simulink library "NeuroMuscularLibrary"  (R2019b)
settings: Solver=ode45  StartTime=0.0  StopTime=10.0  RelTol=1e-3  EnableMultiTasking=on
values from neighbouring files (symbols this model uses):
  a_18_19 = 116    [Prosthesis3R60Params.m]
  a_18_21 = 34    [Prosthesis3R60Params.m]
  a_2_3 = 18    [Prosthesis3R60Params.m]
  angle_offset = 0    [Prosthesis3R60Params.m]
  ankle_height = 0.08    [BodyMechParams.m]
  c = 0.05    [BodyMechParams.m]
  c_jointstop = 0.3 / (pi/180)    (= 17.1887338539)    [BodyMechParams.m]
  c_stance_comp_a0 = 885.0653    [Prosthesis3R60Params.m]
  c_stance_comp_a1 = 2.1443    [Prosthesis3R60Params.m]
  cg14 = 1/2*L14    (= 0.0475)    [Prosthesis3R60Params.m]
  cg25 = (5.45/11.05)*L25    (= 0.0379527149321)    [Prosthesis3R60Params.m]
  cg3 = (3.6/10.4)*L3    (= 0.0306346153846)    [Prosthesis3R60Params.m]
  d_fBall = 0.1    [BodyMechParams.m]
  d_fHeel = 0.05    [BodyMechParams.m]
  deltaLegAngleThr = 8*pi/180    (= 0.13962634016)    [CMGParams.m]
  DeltaThRef = 2e-3    (= 0.002)    [BodyMechParams.m]
  dt_visual = 0.001    [Prosthesis3R60Params.m]
  eref = 0.04    [BodyMechParams.m]
  Fmax = 4000    [MuscleEnergyTest.m]
  FmaxGLU = 1500    [BodyMechParams.m]
  footBallToAnkleDist = 0.16    [BodyMechParams.m]
  footBallToCenterDist = footLength/2    (= 0.1)    [BodyMechParams.m]
  footBallToHeelDist = footLength    (= 0.2)    [BodyMechParams.m]
  footCenterToCGDist = 0.14 - footBallToCenterDist    (= 0.04)    [BodyMechParams.m]
  footInertia = 0.005    [BodyMechParams.m]
  footLength = 0.2    [BodyMechParams.m]
  footMass = 1.25    [BodyMechParams.m]
  FT = 20    [MuscleEnergyTest.m]
  FT_GLU = 47.6    [BodyMechParams.m]
  g = 9.80665    [BodyMechParams.m]
  groundTheta = [atan(diff(groundZ)./diff(groundX)), 0]    [generateGround.m]
  groundZ = groundZ * stepSize/(largestStep+eps)    [generateGround.m]
  hatCenterToCGDist = 0.35 - hatHipToCenterDistLen    (= -0.05)    [BodyMechParams.m]
  hatHipToCenterDistLen = hatLength/2    (= 0.4)    [BodyMechParams.m]
  hatInertia = 3    [BodyMechParams.m]
  hatLeftHipToCenterDistWidth = .15    (= 0.15)    [BodyMechParams.m]
  hatLength = 0.8    [BodyMechParams.m]
  hatMass = 53.5    [BodyMechParams.m]
  hatThickness = 0.2    [BodyMechParams.m]
  hatWidth = 0.4    [BodyMechParams.m]
  J1011 = (4130)*1e-9    (= 4.13e-06)    [Prosthesis3R60Params.m]
  J1415 = (1.18*1e5)*1e-9    (= 0.000118)    [Prosthesis3R60Params.m]
  J18192021 = (6.86*1e4)*1e-9    (= 6.86e-05)    [Prosthesis3R60Params.m]
  J2526 = (3.59*1e4)*1e-9    (= 3.59e-05)    [Prosthesis3R60Params.m]
  J3467 = (25.96*1e4)*1e-9    (= 0.0002596)    [Prosthesis3R60Params.m]
  K = 5    [BodyMechParams.m]
  k_gn = k_gn/2    (= 39226.6)    [BodyMechParams.m]
  k_gt = k_gt/2    (= 39226.6)    [BodyMechParams.m]
  k_pressure = hatMass * g / DeltaThRef    (= 262327.8875)    [BodyMechParams.m]
  k_stance = 130000    [Prosthesis3R60Params.m]
  k_swing = 18750    [Prosthesis3R60Params.m]
  L0_stance = 0.08925    [Prosthesis3R60Params.m]
  L0_swing = 0.0896    [Prosthesis3R60Params.m]
  L10 = 7.9*1e-3    (= 0.0079)    [Prosthesis3R60Params.m]
  L11 = 3.3*1e-3    (= 0.0033)    [Prosthesis3R60Params.m]
  L14 = 95*1e-3    (= 0.095)    [Prosthesis3R60Params.m]
  L15 = 8.2*1e-3    (= 0.0082)    [Prosthesis3R60Params.m]
  L18 = 25.1*1e-3    (= 0.0251)    [Prosthesis3R60Params.m]
  L19 = 17.7*1e-3    (= 0.0177)    [Prosthesis3R60Params.m]
  L20 = 26*1e-3    (= 0.026)    [Prosthesis3R60Params.m]
  L21 = 1.7*1e-3    (= 0.0017)    [Prosthesis3R60Params.m]
  L25 = 76.95*1e-3    (= 0.07695)    [Prosthesis3R60Params.m]
  L26 = 2.8*1e-3    (= 0.0028)    [Prosthesis3R60Params.m]
  L3 = 88.5*1e-3    (= 0.0885)    [Prosthesis3R60Params.m]
  L4 = 1.7*1e-3    (= 0.0017)    [Prosthesis3R60Params.m]
  L6 = 40.25*1e-3    (= 0.04025)    [Prosthesis3R60Params.m]
  L7 = 14.9*1e-3    (= 0.0149)    [Prosthesis3R60Params.m]
  leg_l = [(thighLength - ankle_height/2) (shankLength - ankle_height/2)]    [BodyMechParams.m]
  legAngleSpeedMax = 10    [CMGParams.m]
  lopt = 0.055    [MuscleEnergyTest.m]
  loptBFSH = 0.12    [BodyMechParams.m]
  loptGAS = 0.05    [BodyMechParams.m]
  loptGLU = 0.11    [BodyMechParams.m]
  loptHAB = 0.09    [BodyMechParams.m]
  loptHAD = 0.10    (= 0.1)    [BodyMechParams.m]
  loptHAM = 0.10    (= 0.1)    [BodyMechParams.m]
  loptHFL = 0.11    [BodyMechParams.m]
  loptRF = 0.08    [BodyMechParams.m]
  loptSOL = 0.04    [BodyMechParams.m]
  loptTA = 0.06    [BodyMechParams.m]
  loptVAS = 0.08    [BodyMechParams.m]
  lslack = 0.245    [MuscleEnergyTest.m]
  lslackBFSH = 0.10    (= 0.1)    [BodyMechParams.m]
  lslackGAS = 0.40    (= 0.4)    [BodyMechParams.m]
  lslackGLU = 0.13    [BodyMechParams.m]
  lslackHAB = 0.07    [BodyMechParams.m]
  lslackHAD = 0.18    [BodyMechParams.m]
  lslackHAM = 0.31    [BodyMechParams.m]
  lslackHFL = 0.10    (= 0.1)    [BodyMechParams.m]
  lslackRF = 0.35    [BodyMechParams.m]
  lslackSOL = 0.26    [BodyMechParams.m]
  lslackTA = 0.24    [BodyMechParams.m]
  lslackVAS = 0.23    [BodyMechParams.m]
  m1011 = 49.5*1e-3    (= 0.0495)    [Prosthesis3R60Params.m]
  m1415 = 123.8*1e-3    (= 0.1238)    [Prosthesis3R60Params.m]
  m18192021 = 196.6*1e-3    (= 0.1966)    [Prosthesis3R60Params.m]
  m2526 = 58.3*1e-3    (= 0.0583)    [Prosthesis3R60Params.m]
  m3467 = 253.3*1e-3    (= 0.2533)    [Prosthesis3R60Params.m]
  mu_slide = 0.8    [BodyMechParams.m]
  mu_stick = 0.9    [BodyMechParams.m]
  N = 1.5    [BodyMechParams.m]    (also in cmaes.m = size(x,1); mergeCompareEnergyCosts.m = {S.name})
  phiKneeUpLimit = 5*pi/180    (= 0.0872664625997)    [BodyMechParams.m]
  phimaxGASa = (100-90)*pi/180    (= 0.174532925199)    [BodyMechParams.m]
  phimaxGASk = (180-140)*pi/180    (= 0.698131700798)    [BodyMechParams.m]
  phimaxRFk = (180-165)*pi/180    (= 0.261799387799)    [BodyMechParams.m]
  phimaxSOL = (100-90)*pi/180    (= 0.174532925199)    [BodyMechParams.m]
  phimaxTA = (80-90)*pi/180    (= -0.174532925199)    [BodyMechParams.m]
  phimaxVAS = (180-165)*pi/180    (= 0.261799387799)    [BodyMechParams.m]
  phirefBFSH = (180-160)*pi/180    (= 0.349065850399)    [BodyMechParams.m]
  phirefGASa = (80-90)*pi/180    (= -0.174532925199)    [BodyMechParams.m]
  phirefGASk = (180-165)*pi/180    (= 0.261799387799)    [BodyMechParams.m]
  phirefGLU = (120-180)*pi/180    (= -1.0471975512)    [BodyMechParams.m]
  phirefHAB = 10*pi/180    (= 0.174532925199)    [BodyMechParams.m]
  phirefHAD = 15*pi/180    (= 0.261799387799)    [BodyMechParams.m]
  phirefHAMh = (150-180)*pi/180    (= -0.523598775598)    [BodyMechParams.m]
  phirefHAMk = (180-180)*pi/180    (= 0)    [BodyMechParams.m]
  phirefHFL = (160-180)*pi/180    (= -0.349065850399)    [BodyMechParams.m]
  phirefRFh = (170-180)*pi/180    (= -0.174532925199)    [BodyMechParams.m]
  phirefRFk = (180-125)*pi/180    (= 0.959931088597)    [BodyMechParams.m]
  phirefSOL = (90-90)*pi/180    (= 0)    [BodyMechParams.m]
  ... (+64 more)
undefined symbols (not defined in the file or in its folder): ankleBackDriveGain, ankleCJointstop, ankleDgain, ankleFilterPID, ankleFilterSEA, ankleGearEff, ankleGearRatio, ankleIgain, ankleInitialAngle, ankleInputMass, ankleIntCoulomb, ankleIntDamping, ankleIntStatic, ankleParallelSpringDamping, ankleParallelSpringOffset, ankleParallelSpringStiffness, anklePgain, anklePlantarLimit, ankleSEADamping, ankleSEAStiffness, ankleTendonMass, ankleWMaxJointstop, D12_F, D12_S, D12_T, D12z_T, D13_F, D1G_F, D1G_HAT, D1G_S, D1G_T, D1Gy_F, DeltaS, DeltaSGLU, DeltaSHFL, dryFrictionDamping, dryFrictionStiffness, dryFrictionVelThresh, footMassp, FourBarL1, FourBarL3, GainDphiHATGLUst, GainDphiHATHABst, GainDphiHATHADst, GainDphiHATHFLst, GainFGASst, GainFGLUst, GainFHABst, GainFHAMst, GainFSOLst, GainFSOLTAst, GainFVASst, GainGAS, GainGLU, GainGLUswing, GainHAM, GainHAMHFL ... (+194)
libraries: sm_lib x332, nesl_utility x156, simulink x33, dspswit3 x30, $bdroot x19, simulink_extras x7
(part 4 of 15)

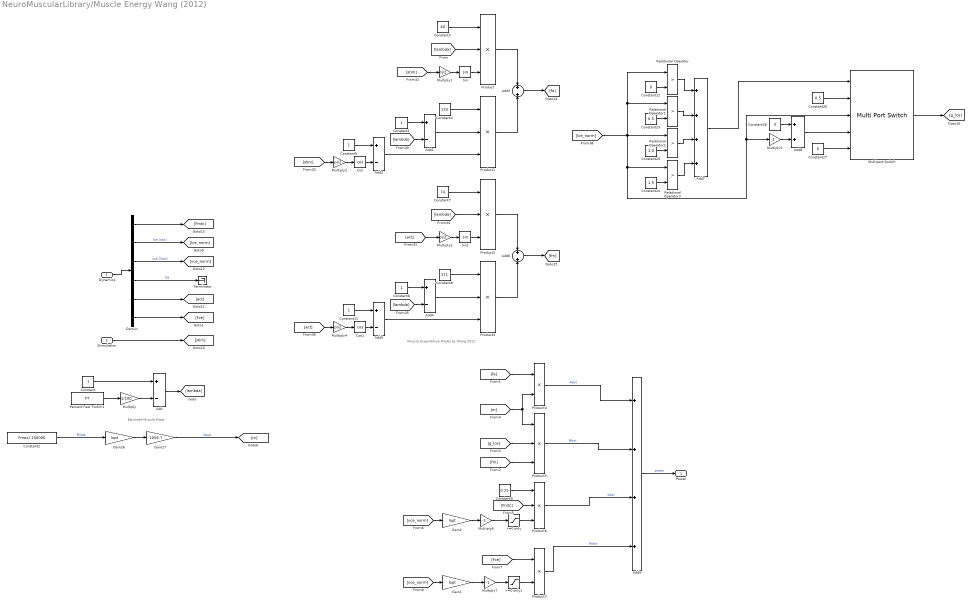
== system NeuroMuscularLibrary/Muscle Energy Wang (2012) ==
  note: Muscle Expenditure Model by Wang 2012
  note: Estimate Muscle Mass
  Dynamics : Inport
  Stimulation : Inport  Port=2
  >=0 only : Saturate  UpperLimit=inf  LowerLimit=0  ZeroCross=off
  >=0 only1 : Saturate  UpperLimit=inf  LowerLimit=0  ZeroCross=off
  Add{,1..2,4..5} (5 alike) : Sum  Inputs=+-
  Add3 : Sum
  Add6 : Sum
  Add7 : Sum  Inputs=++++
  Add8 : Sum
  Add9 : Sum  Inputs=++++
  Constant{,1,5..6,11} (5 alike) : Constant
  Constant12 : Constant  Value=0
  Constant2 : Constant  Value=Fmax/ 250000
  Constant23 : Constant  Value=0.5
  Constant24 : Constant  Value=1.5
  Constant25 : Constant  Value=1.0
  Constant26 : Constant  Value=0.5
  Constant27 : Constant  Value=0
  Constant28 : Constant  Value=3
  Constant3 : Constant  Value=40
  Constant4 : Constant  Value=133
  Constant7 : Constant  Value=74
  Constant8 : Constant  Value=111
  Constant9 : Constant  Value=0.25
  Cos : Trigonometry  Operator=cos
  Cos1 : Trigonometry  Operator=cos
  Demux : Demux  Outputs=6
  Gain1 : Gain  Gain=lopt
  Gain2 : Gain  Gain=lopt
  Gain26 : Gain  Gain=lopt
  Gain27 : Gain  Gain=1059.7
  Multiply : Gain  Gain=1/100
  Multiply{1..4} (4 alike) : Gain  Gain=pi/2
  Multiply5 : Gain  Gain=-2
  Multiply6 : Gain  Gain=-1
  Multiply7 : Gain  Gain=-1
  Multiport Switch : MultiPortSwitch  Inputs=4  DiagnosticForDefault=Warning
  Percent Fast Twitch1 : Constant  Value=FT
  Product{,1..3,5..6} (6 alike) : Product  Inputs=3
  Product4 : Product
  Product7 : Product
  Relational Operator{,1..3} (4 alike) : RelationalOperator  Operator=>  OutDataTypeStr=boolean  RndMeth=Simplest
  Sin : Trigonometry
  Sin1 : Trigonometry
  Terminator : Terminator
  Power : Outport
  wires:
  Demux/6 -> [Fce]
  [vce_norm] -> Gain1/1
  Product7/1 -> Add9/4  "Wdot"
  [Fce] -> Product7/1
  Multiply7/1 -> >=0 only1/1
  Product6/1 -> Add9/3  "Sdot"
  Multiply6/1 -> >=0 only/1
  [vce_norm] -> Gain2/1
  Constant9/1 -> Product6/1
  [Fmtc] -> Product6/2
  Product5/1 -> Add9/2  "Mdot"
  Product4/1 -> Add9/1  "Adot"
  [fm] -> Product5/3
  [g_lce] -> Product5/2
  [fa] -> Product4/1
  [m] -> Product4/2, Product5/1
  Constant2/1 -> Gain26/1  "PCSAL"
  Gain27/1 -> [m]  "Mass"
  Gain26/1 -> Gain27/1
  Multiply5/1 -> Add8/2
  Constant28/1 -> Add8/1
  Add8/1 -> Multiport Switch/4
  Constant27/1 -> Multiport Switch/5
  Constant26/1 -> Multiport Switch/2
  Add7/1 -> Multiport Switch/1
  Relational Operator3/1 -> Add7/4
  Relational Operator2/1 -> Add7/3
  Relational Operator1/1 -> Add7/2
  Relational Operator/1 -> Add7/1
  Constant24/1 -> Relational Operator3/2
  Constant25/1 -> Relational Operator2/2
  Constant23/1 -> Relational Operator1/2
  Constant12/1 -> Relational Operator/2
  [lce_norm] -> Multiport Switch/3, Multiply5/1, Relational Operator3/1, Relational Operator1/1, Relational Operator/1, Relational Operator2/1
  Constant7/1 -> Product2/1
  [act] -> Multiply3/1
  [act] -> Multiply4/1
  [lambda] -> Add4/2
  Cos1/1 -> Add5/2
  Multiply4/1 -> Cos1/1
  Add6/1 -> [fm]
  Constant8/1 -> Product3/1
  [lambda] -> Product2/2
  Add5/1 -> Product3/3
  Add4/1 -> Product3/2
  Multiply3/1 -> Sin1/1
  Constant6/1 -> Add4/1
  Sin1/1 -> Product2/3
  Product2/1 -> Add6/1
  Product3/1 -> Add6/2
  Constant11/1 -> Add5/1
  Cos/1 -> Add2/2
  Add3/1 -> [fa]
  Product/1 -> Add3/1
  Product1/1 -> Add3/2
  Multiply2/1 -> Cos/1
  [stim] -> Multiply2/1
  [stim] -> Multiply1/1
  Multiply1/1 -> Sin/1
  Sin/1 -> Product/3
  Constant5/1 -> Add2/1
  Add2/1 -> Product1/3
  Constant4/1 -> Product1/1
  Add1/1 -> Product1/2
  Constant3/1 -> Product/1
  Constant1/1 -> Add1/1
  [lambda] -> Add1/2
  [lambda] -> Product/2
  Add/1 -> [lambda]
  Multiply/1 -> Add/2
  Percent Fast Twitch1/1 -> Multiply/1
  Constant/1 -> Add/1
  Add9/1 -> Power/1  "power"
  Dynamics/1 -> Demux/1
  Stimulation/1 -> [stim]
  Demux/1 -> [Fmtc]
  Demux/3 -> [vce_norm]  "vce [lopt]"
  Demux/5 -> [act]
  Demux/4 -> Terminator/1  "lse"
  Demux/2 -> [lce_norm]  "lce [opt]"
  >=0 only/1 -> Product6/3
  >=0 only1/1 -> Product7/2
  Multiport Switch/1 -> [g_lce]
  Gain1/1 -> Multiply7/1
  Gain2/1 -> Multiply6/1

== system NeuroMuscularLibrary/Otto-Bock Hydraulic Element ==
  Add : Sum  Commented=on  Inputs=+++
  Add1 : Sum  Inputs=--
  Add2 : Sum  Inputs=+-
  Bumper : Gain  Gain=k
  "Compresion " : Fcn  Commented=on  Expr=u(2)*(u(1)<0)*(u(2)<0)
  Constant1 : Constant  Value=L0
  Constant4 : Constant  Commented=on  Value=0
  Damping coefficient Look-up table : Lookup_n-D  Commented=on  NumberOfTableDimensions=1  BreakpointsForDimension1=dx_points  Table=c  UseLastTableValue=on  InternalRulePriority=Speed  RndMeth=Simplest  InputSameDT=on
  Equal Sign check : Fcn  Expr=u(2)*( (u(1)*u(2)) >0)
  Extension : Fcn  Commented=on  Expr=u(2)*(u(1)>0)*(u(2)>0)
  Force Look-up table : Lookup_n-D  NumberOfTableDimensions=1  BreakpointsForDimension1=dx_points  Table=Fd  UseLastTableValue=on  InternalRulePriority=Speed  RndMeth=Simplest  InputSameDT=on
  Internal Force : sm_lib/Forces and Torques/Internal Force
      settings: SourceProductName=Simscape Multibody  SourceProductBaseCode=MS
  MATLAB Function1 : MATLAB Function  Commented=on  TreatAsAtomicUnit=on
  Multiply1 : Gain  Commented=on
  Multiply2 : Gain  Gain=-1
  Multiply3 : Gain
  Multiply4 : Gain  Gain=-1
  Multiply5 : Gain  Commented=on
  Multiply7 : Gain  Commented=through  Gain=1E6
  Multiply8 : Gain  Commented=through  Gain=1E-6
  Mux : Mux  Inputs=5
  Mux1 : Mux  Commented=on  Inputs=2
  Mux2 : Mux  Commented=on  Inputs=2
  Mux3 : Mux  Inputs=2
  Mux4 : Mux  Commented=on  Inputs=2
  PS-Simulink Converter : nesl_utility/PS-Simulink Converter  PhysicalDomain=network_engine_domain  SubClassName=ps_output  LeftPortType=input  RightPortType=output  PseudoPeriodic=off  Frequencies=[]  Unit=m  AffineConversion=off
  PS-Simulink Converter1 : nesl_utility/PS-Simulink Converter  PhysicalDomain=network_engine_domain  SubClassName=ps_output  LeftPortType=input  RightPortType=output  PseudoPeriodic=off  Frequencies=[]  Unit=m/s  AffineConversion=off
  Product1 : Product  Commented=on
  Round1 : Rounding  Commented=through  Operator=round
  Saturation : Saturate  Commented=on  UpperLimit=inf  LowerLimit=0  ZeroCross=off
  Scope : Scope  Commented=on
  Scope1 : Scope
  Simulink-PS Converter : nesl_utility/Simulink-PS Converter  PhysicalDomain=network_engine_domain  SubClassName=ps_input  LeftPortType=input  RightPortType=output  PseudoPeriodic=off  Frequencies=[]  NoiseDistribution=none  NoiseParameters=[]  Unit=N  AffineConversion=off  FilteringAndDerivatives=provide  SimscapeFilterOrder=1  InputFilterTimeConstant=0.001  UdotUserProvided=0
  Swing Phase Hydraulics : Scope  Commented=on  NumInputPorts=3
  Transform Sensor : sm_lib/Frames and Transforms/Transform Sensor  MeasurementFrame=World  SenseAngle=off  SenseAxis=off  SenseAngle1=off  SenseAngle2=off  SenseAngle3=off  SenseQ=off  SenseR=off  SenseOmegaX=off  SenseOmegaY=off  SenseOmegaZ=off  SenseOmega1=off  SenseOmega2=off  SenseOmega3=off  SenseQDot=off  SenseRDot=off  SenseAlphaX=off  SenseAlphaY=off  SenseAlphaZ=off  SenseAlpha1=off  SenseAlpha2=off  SenseAlpha3=off  SenseQDDot=off  SenseRDDot=off  SenseX=off  SenseY=off  SenseZ=off  SenseRad=off  SenseAzim=off  SenseDist=on  SenseInc=off  SenseXDot=off  SenseYDot=off  SenseZDot=off  SenseRadDot=off  SenseAzimDot=off  SenseDistDot=on  SenseIncDot=off  SenseXDDot=off  SenseYDDot=off  SenseZDDot=off  SenseRadDDot=off  SenseAzimDDot=off  SenseDistDDot=off  SenseIncDDot=off
  c_comp : $bdroot/c  Commented=on  a0=c_comp_a0  a1=c_comp_a1
  c_ext : $bdroot/c  Commented=on  a0=c_ext_a0  a1=c_ext_a1
  Base : PMIOPort  Side=Left
  Follower : PMIOPort  Port=2  Side=Right
  Element info : Outport
  wires:
  Mux/1 -> Element info/1
  PS-Simulink Converter1/1 -> Multiply7/1
  Round1/1 -> Multiply8/1
  Multiply7/1 -> Round1/1
  Multiply3/1 -> Simulink-PS Converter/1, Swing Phase Hydraulics/3, Scope1/1  "F"
  Multiply1/1 -> Mux1/2
  Multiply8/1 -> Swing Phase Hydraulics/2, Mux1/1, Mux/4, Mux2/1, c_ext/1, c_comp/1, Mux3/1, Force Look-up table/1, Mux4/1, Product1/1, Damping coefficient Look-up table/1, MATLAB Function1/2(dx)  "dx"
  Multiply5/1 -> Add/3
  Add2/1 -> Bumper/1, Mux/3  "x"
  "Compresion "/1 -> Add/1
  Extension/1 -> Multiply5/1
  c_comp/1 -> Multiply1/1
  Constant1/1 -> Add2/2
  Equal Sign check/1 -> Add1/1, Multiply4/1  "Fd"
  c_ext/1 -> Mux2/2
  Mux1/1 -> "Compresion "/1
  Add1/1 -> Multiply3/1
  Mux2/1 -> Extension/1
  Constant4/1 -> Add/2
  Bumper/1 -> Add1/2, Multiply2/1  "Fs"
  PS-Simulink Converter/1 -> Swing Phase Hydraulics/1, MATLAB Function1/1(x), Mux/5, Add2/1  "length"
  MATLAB Function1/1(F) -> Scope/1
  Mux3/1 -> Equal Sign check/1
  Force Look-up table/1 -> Mux3/2  "Fd"
  Damping coefficient Look-up table/1 -> Saturation/1  "Fd"
  Mux4/1 -> ?
  Product1/1 -> Mux4/2
  Saturation/1 -> Product1/2
  Multiply2/1 -> Mux/1  "Fs"
  Multiply4/1 -> Mux/2  "Fd"
  connections:
  Transform Sensor/RConn1 -- Follower/RConn1 -- Internal Force/RConn1
  Transform Sensor/RConn3 -- PS-Simulink Converter1/LConn1
  PS-Simulink Converter/LConn1 -- Transform Sensor/RConn2
  Simulink-PS Converter/RConn1 -- Internal Force/LConn2
  Base/RConn1 -- Internal Force/LConn1 -- Transform Sensor/LConn1
